simulink model "fbl_4wd_withCtrller"  (R2020b)
settings: Solver=VariableStepAuto  StartTime=0.0  StopTime=50  RelTol=1e-3
values from neighbouring files (symbols this model uses):
  a = 0.37    [main.m]
  b = 0.55    [main.m]
  d0 = 0.18    [main.m]
  fr_act = 0.12    [main.m]
  g = 9.81    [main.m]
  I = 20    [main.m]
  Ka1 = 0    [main.m]
  Ka2 = 0    [main.m]
  Kp1 = 60    [main.m]
  Kp2 = 60    [main.m]
  Kv1 = 40    [main.m]
  Kv2 = 40    [main.m]
  M = [m 0 0; 0 m 0; 0 0 I]    [main.m]
  m = 116    [main.m]
  mu_act = 0.88    [main.m]
  q0 = [0;0;deg2rad(10)]    [main.m]
  q0_dot = [[cos(q0(3)) -sin(q0(3));sin(q0(3)) cos(q0(3))]*[0.5;0.5];-2.2]    [main.m]
  r = 0.2    [main.m]
settings Model: Creator=sumit  LastModifiedBy=sumit
settings SolverCC: AlgebraicLoopSolver=LineSearch

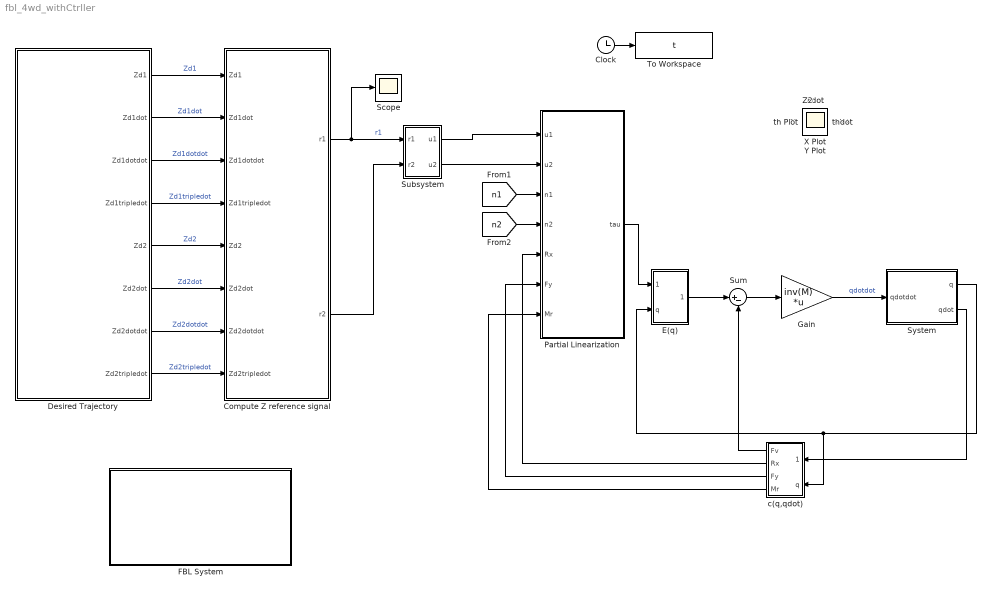
== system fbl_4wd_withCtrller ==
  Clock : Clock
  Compute Z reference signal : Subsystem
  Desired Trajectory : Subsystem
  E(q) : Subsystem
  FBL System : Subsystem
  Gain : Gain  Gain=inv(M)  Multiplication=Matrix(K*u)
  Partial Linearization : MATLAB Function  TreatAsAtomicUnit=on
      settings: MinAlgLoopOccurrences=on
  Scope : Scope
  Subsystem : Subsystem
  Sum : Sum  Inputs=|+-
  System : Subsystem
  To Workspace : ToWorkspace  VariableName=t  SampleTime=-1
  c(q,qdot) : Subsystem
  X Plot : Scope
  Xdot : Scope
  Y Plot : Scope
  Ydot : Scope
  Z1 : Scope
  Z2 : Scope
  th Plot : Scope
  thdot : Scope
  wires:
  Clock/1 -> To Workspace/1
  Sum/1 -> Gain/1
  c(q,qdot)/1(Fv) -> Sum/2
  E(q)/1(Ftau) -> Sum/1
  Partial Linearization/1(tau) -> E(q)/1(tau)
  c(q,qdot)/4(Mr) -> Partial Linearization/7(Mr)
  c(q,qdot)/3(Fy) -> Partial Linearization/6(Fy)
  c(q,qdot)/2(Rx) -> Partial Linearization/5(Rx)
  [n1] -> Partial Linearization/3(n1)
  [n2] -> Partial Linearization/4(n2)
  Desired Trajectory/1(Zd1) -> Compute Z reference signal/1(Zd1)  "Zd1"
  Desired Trajectory/2(Zd1dot) -> Compute Z reference signal/2(Zd1dot)  "Zd1dot"
  Desired Trajectory/3(Zd1dotdot) -> Compute Z reference signal/3(Zd1dotdot)  "Zd1dotdot"
  Desired Trajectory/4(Zd1tripledot) -> Compute Z reference signal/4(Zd1tripledot)  "Zd1tripledot"
  Desired Trajectory/5(Zd2) -> Compute Z reference signal/5(Zd2)  "Zd2"
  Desired Trajectory/6(Zd2dot) -> Compute Z reference signal/6(Zd2dot)  "Zd2dot"
  Desired Trajectory/7(Zd2dotdot) -> Compute Z reference signal/7(Zd2dotdot)  "Zd2dotdot"
  Desired Trajectory/8(Zd2tripledot) -> Compute Z reference signal/8(Zd2tripledot)  "Zd2tripledot"
  Compute Z reference signal/1(r1) -> Scope/1, Subsystem/1(r1)  "r1"
  Compute Z reference signal/2(r2) -> Subsystem/2(r2)
  Subsystem/1(u1) -> Partial Linearization/1(u1)
  Subsystem/2(u2) -> Partial Linearization/2(u2)
  System/1(q) -> c(q,qdot)/2(q), E(q)/2(q)
  Gain/1 -> System/1(qdotdot)  "qdotdot"
  System/2(qdot) -> c(q,qdot)/1(qdot)

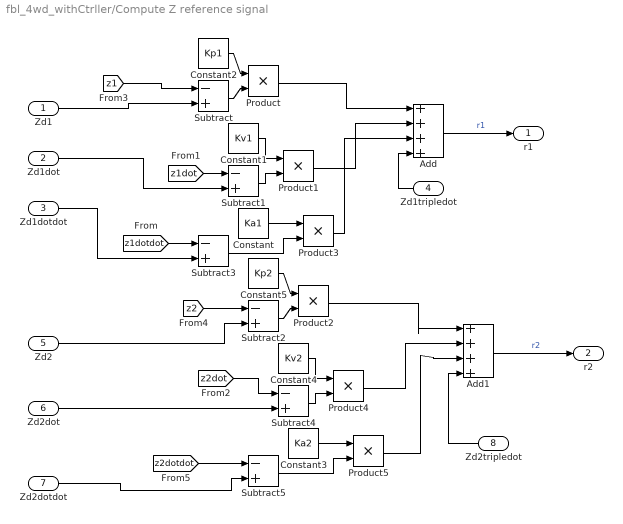
== system fbl_4wd_withCtrller/Compute Z reference signal ==
  Zd1 : Inport
  Zd1dot : Inport  Port=2
  Zd1dotdot : Inport  Port=3
  Zd1tripledot : Inport  Port=4
  Zd2 : Inport  Port=5
  Zd2dot : Inport  Port=6
  Zd2dotdot : Inport  Port=7
  Zd2tripledot : Inport  Port=8
  Add : Sum  Inputs=++++
  Add1 : Sum  Inputs=++++
  Constant : Constant  Value=Ka1
  Constant1 : Constant  Value=Kv1
  Constant2 : Constant  Value=Kp1
  Constant3 : Constant  Value=Ka2
  Constant4 : Constant  Value=Kv2
  Constant5 : Constant  Value=Kp2
  Product{,1..5} (6 alike) : Product
  Subtract{,1..5} (6 alike) : Sum  Inputs=-+
  r1 : Outport
  r2 : Outport  Port=2
  wires:
  Zd2dot/1 -> Subtract4/2
  Constant5/1 -> Product2/1
  [z2] -> Subtract2/1
  Product/1 -> Add/1
  Product3/1 -> Add/3
  Subtract1/1 -> Product1/2
  [z2dot] -> Subtract4/1
  Subtract4/1 -> Product4/2
  Subtract5/1 -> Product5/2
  Product5/1 -> Add1/3
  Constant2/1 -> Product/1
  Zd1/1 -> Subtract/2
  Product2/1 -> Add1/1
  Add1/1 -> r2/1  "r2"
  Product4/1 -> Add1/2
  Subtract3/1 -> Product3/2
  Constant4/1 -> Product4/1
  Constant3/1 -> Product5/1
  Add/1 -> r1/1  "r1"
  Subtract2/1 -> Product2/2
  [z1dot] -> Subtract1/1
  Constant1/1 -> Product1/1
  Zd1dot/1 -> Subtract1/2
  Constant/1 -> Product3/1
  Subtract/1 -> Product/2
  Product1/1 -> Add/2
  [z2dotdot] -> Subtract5/1
  Zd1tripledot/1 -> Add/4
  Zd1dotdot/1 -> Subtract3/2
  [z1] -> Subtract/1
  Zd2tripledot/1 -> Add1/4
  [z1dotdot] -> Subtract3/1
  Zd2dotdot/1 -> Subtract5/2
  Zd2/1 -> Subtract2/2

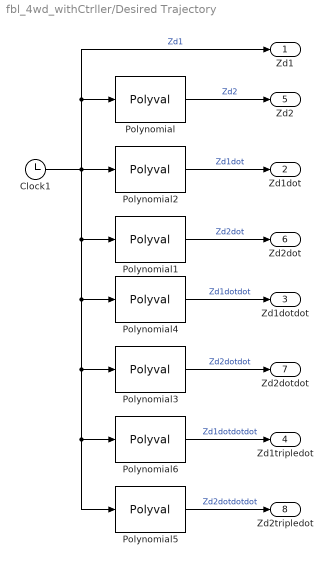
== system fbl_4wd_withCtrller/Desired Trajectory ==
  Clock1 : Clock
  Polynomial : Polyval  Coefs=[-0.002 0.1 0.1 0]
  Polynomial1 : Polyval  Coefs=[-0.006 0.2 0.1]
  Polynomial2 : Polyval  Coefs=[1]
  Polynomial3 : Polyval  Coefs=[-0.012 0.2]
  Polynomial4 : Polyval  Coefs=[0]
  Polynomial5 : Polyval  Coefs=[-0.012 0.2]
  Polynomial6 : Polyval  Coefs=[0]
  Zd1 : Outport
  Zd1dot : Outport  Port=2
  Zd1dotdot : Outport  Port=3
  Zd1tripledot : Outport  Port=4
  Zd2 : Outport  Port=5
  Zd2dot : Outport  Port=6
  Zd2dotdot : Outport  Port=7
  Zd2tripledot : Outport  Port=8
  wires:
  Polynomial/1 -> Zd2/1  "Zd2"
  Polynomial1/1 -> Zd2dot/1  "Zd2dot"
  Polynomial2/1 -> Zd1dot/1  "Zd1dot"
  Polynomial4/1 -> Zd1dotdot/1  "Zd1dotdot"
  Polynomial3/1 -> Zd2dotdot/1  "Zd2dotdot"
  Polynomial6/1 -> Zd1tripledot/1  "Zd1dotdotdot"
  Polynomial5/1 -> Zd2tripledot/1  "Zd2dotdotdot"
  Clock1/1 -> Polynomial6/1, Polynomial5/1, Polynomial3/1, Polynomial4/1, Polynomial1/1, Polynomial2/1, Zd1/1, Polynomial/1  "Zd1"

== system fbl_4wd_withCtrller/E(q) ==
  tau : Inport
  q : Inport  Port=2
  Demux : Demux  Outputs=3
  Eq : MATLAB Function  TreatAsAtomicUnit=on
      settings: MinAlgLoopOccurrences=on
  Terminator : Terminator
  Terminator1 : Terminator
  Ftau : Outport
  wires:
  Demux/1 -> Terminator/1
  Eq/1(Ftau) -> Ftau/1
  q/1 -> Demux/1
  Demux/2 -> Terminator1/1
  tau/1 -> Eq/1(tau)
  Demux/3 -> Eq/2(theta)

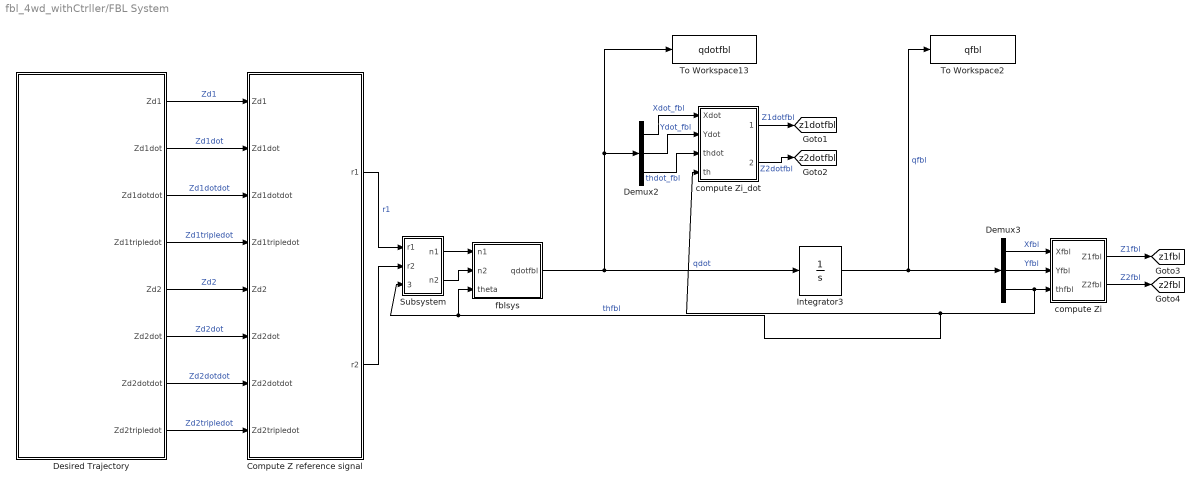
== system fbl_4wd_withCtrller/FBL System ==
  Compute Z reference signal : Subsystem
  Demux2 : Demux  Outputs=3
  Demux3 : Demux  Outputs=3
  Desired Trajectory : Subsystem
  Integrator3 : Integrator  InitialCondition=q0
  Subsystem : Subsystem
  To Workspace13 : ToWorkspace  VariableName=qdotfbl  SampleTime=-1
  To Workspace2 : ToWorkspace  VariableName=qfbl  SampleTime=-1
  compute Zi : Subsystem
  compute Zi_dot : Subsystem
  fblsys : MATLAB Function  TreatAsAtomicUnit=on
  tag scope: z1dotfbl=global, z1fbl=global, z2dotfbl=global, z2fbl=global
  wires:
  Integrator3/1 -> Demux3/1, To Workspace2/1  "qfbl"
  fblsys/1(qdotfbl) -> Integrator3/1, To Workspace13/1, Demux2/1  "qdot"
  Demux3/3 -> fblsys/3(theta), Subsystem/3(theta), compute Zi_dot/4(th), compute Zi/3(thfbl)  "thfbl"
  Demux2/1 -> compute Zi_dot/1(Xdot)  "Xdot_fbl"
  Demux2/3 -> compute Zi_dot/3(thdot)  "thdot_fbl"
  Demux2/2 -> compute Zi_dot/2(Ydot)  "Ydot_fbl"
  Demux3/1 -> compute Zi/1(Xfbl)  "Xfbl"
  Demux3/2 -> compute Zi/2(Yfbl)  "Yfbl"
  compute Zi/1(Z1fbl) -> [z1fbl]  "Z1fbl"
  compute Zi/2(Z2fbl) -> [z2fbl]  "Z2fbl"
  Desired Trajectory/2(Zd1dot) -> Compute Z reference signal/2(Zd1dot)  "Zd1dot"
  Desired Trajectory/7(Zd2dotdot) -> Compute Z reference signal/7(Zd2dotdot)  "Zd2dotdot"
  Desired Trajectory/6(Zd2dot) -> Compute Z reference signal/6(Zd2dot)  "Zd2dot"
  Desired Trajectory/3(Zd1dotdot) -> Compute Z reference signal/3(Zd1dotdot)  "Zd1dotdot"
  Desired Trajectory/5(Zd2) -> Compute Z reference signal/5(Zd2)  "Zd2"
  Desired Trajectory/8(Zd2tripledot) -> Compute Z reference signal/8(Zd2tripledot)  "Zd2tripledot"
  Desired Trajectory/4(Zd1tripledot) -> Compute Z reference signal/4(Zd1tripledot)  "Zd1tripledot"
  Desired Trajectory/1(Zd1) -> Compute Z reference signal/1(Zd1)  "Zd1"
  Compute Z reference signal/1(r1) -> Subsystem/1(r1)  "r1"
  Compute Z reference signal/2(r2) -> Subsystem/2(r2)
  Subsystem/2(n2) -> fblsys/2(n2)
  Subsystem/1(n1) -> fblsys/1(n1)
  compute Zi_dot/1(Z1dot) -> [z1dotfbl]  "Z1dotfbl"
  compute Zi_dot/2(Z2dot) -> [z2dotfbl]  "Z2dotfbl"

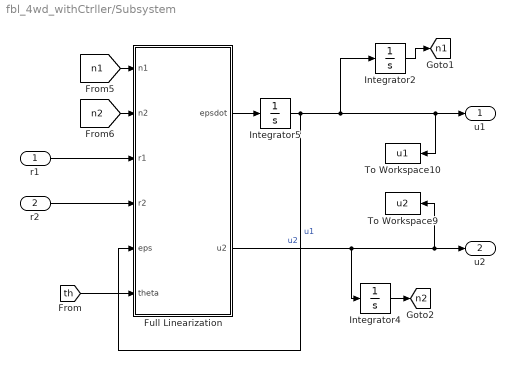
== system fbl_4wd_withCtrller/Subsystem ==
  r1 : Inport
  r2 : Inport  Port=2
  Full Linearization : MATLAB Function  TreatAsAtomicUnit=on
      settings: MinAlgLoopOccurrences=on
  Integrator2 : Integrator
  Integrator4 : Integrator
  Integrator5 : Integrator
  To Workspace10 : ToWorkspace  VariableName=u1  SampleTime=-1
  To Workspace9 : ToWorkspace  VariableName=u2  SampleTime=-1
  u1 : Outport
  u2 : Outport  Port=2
  tag scope: n1=global, n2=global
  wires:
  [n1] -> Full Linearization/1(n1)
  Full Linearization/1(epsdot) -> Integrator5/1
  Full Linearization/2(u2) -> Integrator4/1, To Workspace9/1, u2/1  "u2"
  Integrator5/1 -> Integrator2/1, u1/1, To Workspace10/1, Full Linearization/5(eps)  "u1"
  [n2] -> Full Linearization/2(n2)
  r1/1 -> Full Linearization/3(r1)
  Integrator2/1 -> [n1]
  Integrator4/1 -> [n2]
  [th] -> Full Linearization/6(theta)
  r2/1 -> Full Linearization/4(r2)

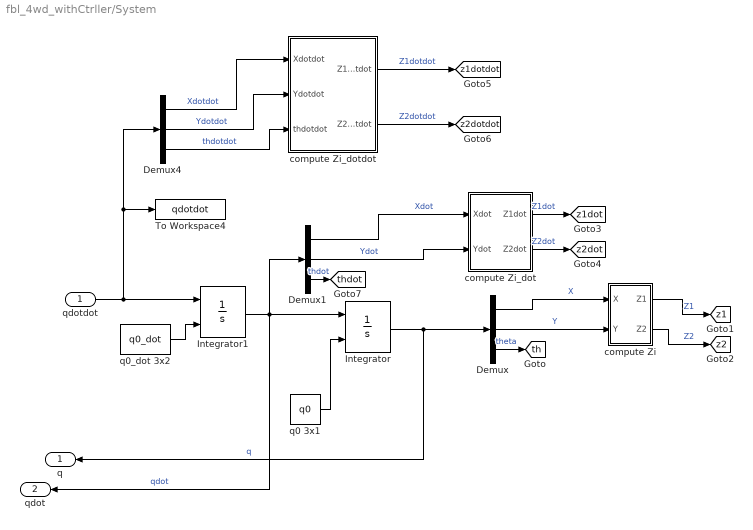
== system fbl_4wd_withCtrller/System ==
  qdotdot : Inport
  Demux : Demux  Outputs=3
  Demux1 : Demux  Outputs=3
  Demux4 : Demux  Outputs=3
  Integrator : Integrator  InitialConditionSource=external
  Integrator1 : Integrator  InitialConditionSource=external
  To Workspace4 : ToWorkspace  VariableName=qdotdot  SampleTime=-1
  compute Zi : Subsystem
  compute Zi_dot : Subsystem
  compute Zi_dotdot : Subsystem
  q0 3x1 : Constant  Value=q0
  q0_dot 3x2 : Constant  Value=q0_dot
  q : Outport
  qdot : Outport  Port=2
  tag scope: th=global, thdot=global, z1=global, z1dot=global, z1dotdot=global, z2=global, z2dot=global, z2dotdot=global
  wires:
  compute Zi_dot/2(Z2dot) -> [z2dot]  "Z2dot"
  Demux1/3 -> [thdot]  "thdot"
  Demux/3 -> [th]  "theta"
  Demux4/2 -> compute Zi_dotdot/2(Ydotdot)  "Ydotdot"
  qdotdot/1 -> Integrator1/1, Demux4/1, To Workspace4/1
  q0_dot 3x2/1 -> Integrator1/2
  Demux4/3 -> compute Zi_dotdot/3(thdotdot)  "thdotdot"
  compute Zi/2(Z2) -> [z2]  "Z2"
  q0 3x1/1 -> Integrator/2
  compute Zi_dotdot/1(Z1dotdot) -> [z1dotdot]  "Z1dotdot"
  Integrator/1 -> q/1, Demux/1  "q"
  Demux1/2 -> compute Zi_dot/2(Ydot)  "Ydot"
  Integrator1/1 -> qdot/1, Demux1/1, Integrator/1  "qdot"
  compute Zi_dotdot/2(Z2dotdot) -> [z2dotdot]  "Z2dotdot"
  compute Zi/1(Z1) -> [z1]  "Z1"
  Demux/1 -> compute Zi/1(X)  "X"
  Demux1/1 -> compute Zi_dot/1(Xdot)  "Xdot"
  Demux/2 -> compute Zi/2(Y)  "Y"
  compute Zi_dot/1(Z1dot) -> [z1dot]  "Z1dot"
  Demux4/1 -> compute Zi_dotdot/1(Xdotdot)  "Xdotdot"

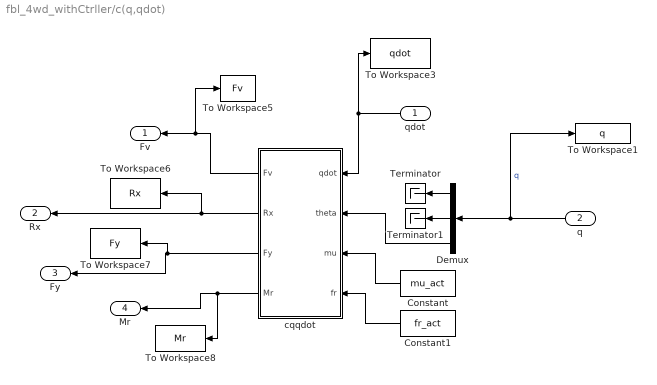
== system fbl_4wd_withCtrller/c(q,qdot) ==
  qdot : Inport
  q : Inport  Port=2
  Constant : Constant  Value=mu_act
  Constant1 : Constant  Value=fr_act
  Demux : Demux  Outputs=3
  Terminator : Terminator
  Terminator1 : Terminator
  To Workspace1 : ToWorkspace  VariableName=q  SampleTime=-1
  To Workspace3 : ToWorkspace  VariableName=qdot  SampleTime=-1
  To Workspace5 : ToWorkspace  VariableName=Fv  SampleTime=-1
  To Workspace6 : ToWorkspace  VariableName=Rx  SampleTime=-1
  To Workspace7 : ToWorkspace  VariableName=Fy  SampleTime=-1
  To Workspace8 : ToWorkspace  VariableName=Mr  SampleTime=-1
  cqqdot : MATLAB Function  TreatAsAtomicUnit=on
  Fv : Outport
  Rx : Outport  Port=2
  Fy : Outport  Port=3
  Mr : Outport  Port=4
  wires:
  Demux/2 -> Terminator1/1
  qdot/1 -> To Workspace3/1, cqqdot/1(qdot)
  Constant1/1 -> cqqdot/4(fr)
  Demux/1 -> Terminator/1
  Constant/1 -> cqqdot/3(mu)
  Demux/3 -> cqqdot/2(theta)
  cqqdot/3(Fy) -> To Workspace7/1, Fy/1
  cqqdot/2(Rx) -> To Workspace6/1, Rx/1
  cqqdot/4(Mr) -> To Workspace8/1, Mr/1
  cqqdot/1(Fv) -> To Workspace5/1, Fv/1
  q/1 -> To Workspace1/1, Demux/1  "q"

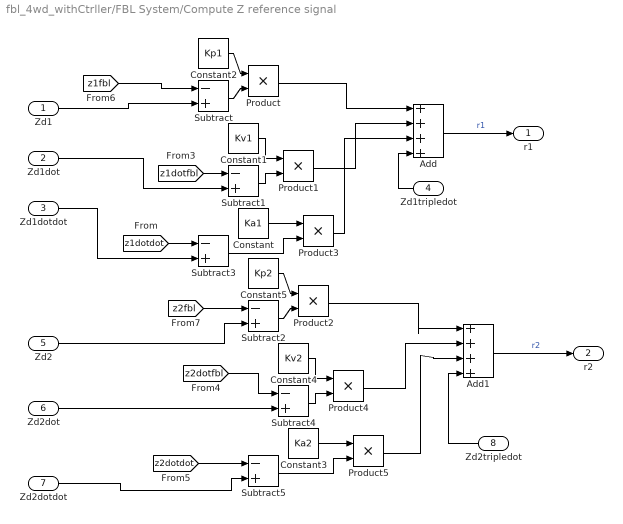
== system fbl_4wd_withCtrller/FBL System/Compute Z reference signal ==
  Zd1 : Inport
  Zd1dot : Inport  Port=2
  Zd1dotdot : Inport  Port=3
  Zd1tripledot : Inport  Port=4
  Zd2 : Inport  Port=5
  Zd2dot : Inport  Port=6
  Zd2dotdot : Inport  Port=7
  Zd2tripledot : Inport  Port=8
  Add : Sum  Inputs=++++
  Add1 : Sum  Inputs=++++
  Constant : Constant  Value=Ka1
  Constant1 : Constant  Value=Kv1
  Constant2 : Constant  Value=Kp1
  Constant3 : Constant  Value=Ka2
  Constant4 : Constant  Value=Kv2
  Constant5 : Constant  Value=Kp2
  Product{,1..5} (6 alike) : Product
  Subtract{,1..5} (6 alike) : Sum  Inputs=-+
  r1 : Outport
  r2 : Outport  Port=2
  wires:
  Zd2dot/1 -> Subtract4/2
  Constant5/1 -> Product2/1
  [z2fbl] -> Subtract2/1
  Product/1 -> Add/1
  Product3/1 -> Add/3
  Subtract1/1 -> Product1/2
  [z2dotfbl] -> Subtract4/1
  Subtract4/1 -> Product4/2
  Subtract5/1 -> Product5/2
  Product5/1 -> Add1/3
  Constant2/1 -> Product/1
  Zd1/1 -> Subtract/2
  Product2/1 -> Add1/1
  Add1/1 -> r2/1  "r2"
  Product4/1 -> Add1/2
  Subtract3/1 -> Product3/2
  Constant4/1 -> Product4/1
  Constant3/1 -> Product5/1
  Add/1 -> r1/1  "r1"
  Subtract2/1 -> Product2/2
  [z1dotfbl] -> Subtract1/1
  Constant1/1 -> Product1/1
  Zd1dot/1 -> Subtract1/2
  Constant/1 -> Product3/1
  Subtract/1 -> Product/2
  Product1/1 -> Add/2
  [z2dotdot] -> Subtract5/1
  Zd1tripledot/1 -> Add/4
  Zd1dotdot/1 -> Subtract3/2
  [z1fbl] -> Subtract/1
  Zd2tripledot/1 -> Add1/4
  [z1dotdot] -> Subtract3/1
  Zd2dotdot/1 -> Subtract5/2
  Zd2/1 -> Subtract2/2

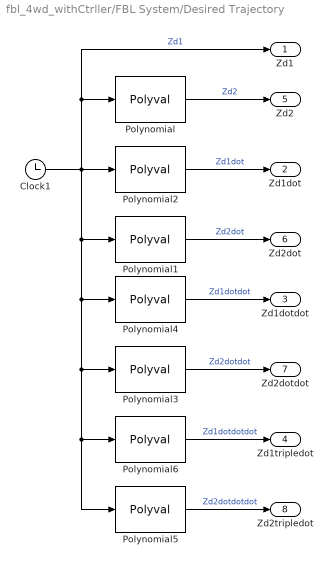
== system fbl_4wd_withCtrller/FBL System/Desired Trajectory ==
  Clock1 : Clock
  Polynomial : Polyval  Coefs=[-0.002 0.1 0.1 0]
  Polynomial1 : Polyval  Coefs=[-0.006 0.2 0.1]
  Polynomial2 : Polyval  Coefs=[1]
  Polynomial3 : Polyval  Coefs=[-0.012 0.2]
  Polynomial4 : Polyval  Coefs=[0]
  Polynomial5 : Polyval  Coefs=[-0.012 0.2]
  Polynomial6 : Polyval  Coefs=[0]
  Zd1 : Outport
  Zd1dot : Outport  Port=2
  Zd1dotdot : Outport  Port=3
  Zd1tripledot : Outport  Port=4
  Zd2 : Outport  Port=5
  Zd2dot : Outport  Port=6
  Zd2dotdot : Outport  Port=7
  Zd2tripledot : Outport  Port=8
  wires:
  Polynomial/1 -> Zd2/1  "Zd2"
  Polynomial1/1 -> Zd2dot/1  "Zd2dot"
  Polynomial2/1 -> Zd1dot/1  "Zd1dot"
  Polynomial4/1 -> Zd1dotdot/1  "Zd1dotdot"
  Polynomial3/1 -> Zd2dotdot/1  "Zd2dotdot"
  Polynomial6/1 -> Zd1tripledot/1  "Zd1dotdotdot"
  Polynomial5/1 -> Zd2tripledot/1  "Zd2dotdotdot"
  Clock1/1 -> Polynomial6/1, Polynomial5/1, Polynomial3/1, Polynomial4/1, Polynomial1/1, Polynomial2/1, Zd1/1, Polynomial/1  "Zd1"

== system fbl_4wd_withCtrller/FBL System/Subsystem ==
  r1 : Inport
  r2 : Inport  Port=2
  theta : Inport  Port=3
  Full Linearization : MATLAB Function  TreatAsAtomicUnit=on
      settings: MinAlgLoopOccurrences=on
  Integrator2 : Integrator
  Integrator4 : Integrator
  Integrator5 : Integrator
  To Workspace1 : ToWorkspace  VariableName=n1fbl  SampleTime=-1
  To Workspace10 : ToWorkspace  VariableName=u1fbl  SampleTime=-1
  To Workspace2 : ToWorkspace  VariableName=n2fbl  SampleTime=-1
  To Workspace9 : ToWorkspace  VariableName=u2fbl  SampleTime=-1
  n1 : Outport
  n2 : Outport  Port=2
  wires:
  Integrator2/1 -> To Workspace1/1, Full Linearization/1(n1), n1/1
  Full Linearization/1(epsdot) -> Integrator5/1
  Full Linearization/2(u2) -> Integrator4/1, To Workspace9/1  "u2"
  Integrator5/1 -> Integrator2/1, To Workspace10/1, Full Linearization/5(eps)  "u1"
  Integrator4/1 -> To Workspace2/1, Full Linearization/2(n2), n2/1
  r1/1 -> Full Linearization/3(r1)
  theta/1 -> Full Linearization/6(theta)
  r2/1 -> Full Linearization/4(r2)

== system fbl_4wd_withCtrller/FBL System/compute Zi ==
  Xfbl : Inport
  Yfbl : Inport  Port=2
  thfbl : Inport  Port=3
  Constant : Constant  Value=d0
  Constant1 : Constant  Value=d0
  Cos : Trigonometry  Operator=cos
  Cos1 : Trigonometry
  Product : Product
  Product1 : Product
  Sum1 : Sum
  Sum2 : Sum
  Z1fbl : Outport
  Z2fbl : Outport  Port=2
  wires:
  Product1/1 -> Sum2/2
  Cos1/1 -> Product1/1
  Cos/1 -> Product/1
  Xfbl/1 -> Sum1/1
  Constant1/1 -> Product1/2
  thfbl/1 -> Cos1/1, Cos/1
  Product/1 -> Sum1/2
  Constant/1 -> Product/2
  Yfbl/1 -> Sum2/1
  Sum1/1 -> Z1fbl/1  "Z1fbl"
  Sum2/1 -> Z2fbl/1  "Z2fbl"

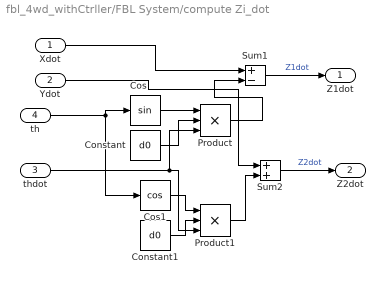
== system fbl_4wd_withCtrller/FBL System/compute Zi_dot ==
  Xdot : Inport
  Ydot : Inport  Port=2
  thdot : Inport  Port=3
  th : Inport  Port=4
  Constant : Constant  Value=d0
  Constant1 : Constant  Value=d0
  Cos : Trigonometry
  Cos1 : Trigonometry  Operator=cos
  Product : Product  Inputs=3
  Product1 : Product  Inputs=3
  Sum1 : Sum  Inputs=+-
  Sum2 : Sum
  Z1dot : Outport
  Z2dot : Outport  Port=2
  wires:
  Product1/1 -> Sum2/2
  Cos1/1 -> Product1/1
  Cos/1 -> Product/1
  Xdot/1 -> Sum1/1
  Constant1/1 -> Product1/2
  th/1 -> Cos1/1, Cos/1
  Product/1 -> Sum1/2
  Constant/1 -> Product/2
  Ydot/1 -> Sum2/1
  Sum1/1 -> Z1dot/1  "Z1dot"
  Sum2/1 -> Z2dot/1  "Z2dot"
  thdot/1 -> Product/3, Product1/3

== system fbl_4wd_withCtrller/System/compute Zi ==
  X : Inport
  Y : Inport  Port=2
  Constant : Constant  Value=d0
  Constant1 : Constant  Value=d0
  Cos : Trigonometry  Operator=cos
  Cos1 : Trigonometry
  Product : Product
  Product1 : Product
  Sum1 : Sum
  Sum2 : Sum
  Z1 : Outport
  Z2 : Outport  Port=2
  wires:
  Product1/1 -> Sum2/2
  Cos1/1 -> Product1/1
  Cos/1 -> Product/1
  X/1 -> Sum1/1
  Constant1/1 -> Product1/2
  [th] -> Cos/1, Cos1/1
  Product/1 -> Sum1/2
  Constant/1 -> Product/2
  Y/1 -> Sum2/1
  Sum1/1 -> Z1/1  "Z1"
  Sum2/1 -> Z2/1  "Z2"

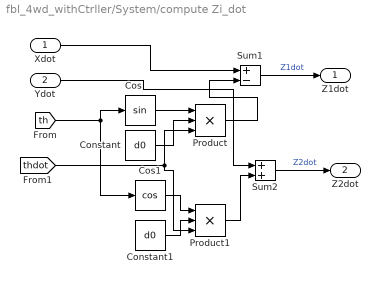
== system fbl_4wd_withCtrller/System/compute Zi_dot ==
  Xdot : Inport
  Ydot : Inport  Port=2
  Constant : Constant  Value=d0
  Constant1 : Constant  Value=d0
  Cos : Trigonometry
  Cos1 : Trigonometry  Operator=cos
  Product : Product  Inputs=3
  Product1 : Product  Inputs=3
  Sum1 : Sum  Inputs=+-
  Sum2 : Sum
  Z1dot : Outport
  Z2dot : Outport  Port=2
  wires:
  Product1/1 -> Sum2/2
  Cos1/1 -> Product1/1
  Cos/1 -> Product/1
  Xdot/1 -> Sum1/1
  Constant1/1 -> Product1/2
  [th] -> Cos/1, Cos1/1
  Product/1 -> Sum1/2
  Constant/1 -> Product/2
  Ydot/1 -> Sum2/1
  Sum1/1 -> Z1dot/1  "Z1dot"
  Sum2/1 -> Z2dot/1  "Z2dot"
  [thdot] -> Product1/3, Product/3

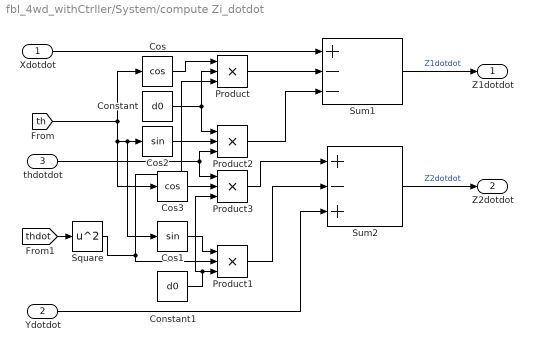
== system fbl_4wd_withCtrller/System/compute Zi_dotdot ==
  Xdotdot : Inport
  Ydotdot : Inport  Port=2
  thdotdot : Inport  Port=3
  Constant : Constant  Value=d0
  Constant1 : Constant  Value=d0
  Cos : Trigonometry  Operator=cos
  Cos1 : Trigonometry
  Cos2 : Trigonometry
  Cos3 : Trigonometry  Operator=cos
  Product{,1..3} (4 alike) : Product  Inputs=3
  Square : Math  Operator=square  SaturateOnIntegerOverflow=on
  Sum1 : Sum  Inputs=+--
  Sum2 : Sum  Inputs=+-+
  Z1dotdot : Outport
  Z2dotdot : Outport  Port=2
  wires:
  Product1/1 -> Sum2/2
  Cos1/1 -> Product1/1
  Cos/1 -> Product/1
  Xdotdot/1 -> Sum1/1
  [th] -> Cos3/1, Cos2/1, Cos1/1, Cos/1
  Product/1 -> Sum1/2
  Constant/1 -> Product2/1, Product/2
  Sum1/1 -> Z1dotdot/1  "Z1dotdot"
  Sum2/1 -> Z2dotdot/1  "Z2dotdot"
  [thdot] -> Square/1
  Square/1 -> Product/3, Product1/2
  Cos2/1 -> Product2/2
  thdotdot/1 -> Product3/1, Product2/3
  Ydotdot/1 -> Sum2/3
  Constant1/1 -> Product3/3, Product1/3
  Product2/1 -> Sum1/3
  Product3/1 -> Sum2/1
  Cos3/1 -> Product3/2

== matlab function fbl_4wd_withCtrller/E(q)/Eq ==
  data: tau input; theta input; Ftau output; t parameter; r parameter
function Ftau = Eq(tau,theta,t, r)
Ftau=[cos(theta)/r cos(theta)/r;...
   sin(theta)/r sin(theta)/r;...
   -t/r t/r]*tau;

== matlab function fbl_4wd_withCtrller/c(q,qdot)/cqqdot ==
  data: qdot input; theta input; Fv output; mu input; fr input; a parameter; b parameter; t parameter; g parameter; m parameter; Rx output; Fy output; Mr output
function [Fv,Rx,Fy,Mr] = cqqdot(qdot,theta,mu,fr,a, b, t, g, m)
Xdot=qdot(1);
Ydot=qdot(2);
thdot=qdot(3);

%Rth = [cos(theta) -sin(theta);sin(theta) cos(theta)];

xdot =  Xdot*cos(theta)+Ydot*sin(theta);
ydot = -Xdot*sin(theta)+Ydot*cos(theta);

x1dot = xdot-t*thdot;   
x2dot = xdot+t*thdot;
y1dot = ydot+a*thdot;
y3dot = ydot-b*thdot;

Rx = fr*m*g*0.5*(sign(x1dot)+sign(x2dot));
Fy = mu*m*g*(b*sign(y1dot)+a*sign(y3dot))/(a+b);
Mr = mu*a*b*m*g*(sign(y1dot)-sign(y3dot))/(a+b)...
     + fr*t*m*g*0.5*(sign(x2dot)-sign(x1dot));
 
Fv=[Rx*cos(theta)-Fy*sin(theta);...
   Rx*sin(theta)+Fy*cos(theta);...
   Mr];

== matlab function fbl_4wd_withCtrller/Partial Linearization ==
  data: u1 input; u2 input; n1 input; n2 input; Rx input; Fy input; Mr input; tau output; t parameter; r parameter; d0 parameter; m parameter; I parameter
function tau = FBL(u1,u2,n1,n2,Rx,Fy,Mr,t, r,d0, m, I)
tau=[r*0.5*(m*u1+m*n2*n2/d0+Rx)+(r*d0*0.5/t)*((m+I/(d0^2))*u2-m*n1*n2/d0...
    +Fy-Mr/d0);
     r*0.5*(m*u1+m*n2*n2/d0+Rx)-(r*d0*0.5/t)*((m+I/(d0^2))*u2-m*n1*n2/d0...
    +Fy-Mr/d0)];

== matlab function fbl_4wd_withCtrller/FBL System/fblsys ==
  data: n1 input; n2 input; theta input; qdotfbl output; d0 parameter
function qdotfbl = fblsys(n1, n2,theta,d0)
qdotfbl=[cos(theta)*n1-sin(theta)*n2;...
         sin(theta)*n1+cos(theta)*n2;...
         -n2/d0];

== matlab function fbl_4wd_withCtrller/Subsystem/Full Linearization ==
  data: n1 input; n2 input; d0 parameter; r1 input; r2 input; eps input; theta input; epsdot output; u2 output
function [epsdot,u2] = fulllin(n1,n2,d0,r1,r2, eps,theta)
epsdot = cos(theta)*r1+sin(theta)*r2+n1*n2*n2/(d0^2);
if round(n1)==0
    u2=0;
else
u2 = (sin(theta)*r1-cos(theta)*r2)*d0/n1-2*eps*n2/n1;
end

== matlab function fbl_4wd_withCtrller/FBL System/Subsystem/Full Linearization ==
  data: n1 input; n2 input; d0 parameter; r1 input; r2 input; eps input; theta input; epsdot output; u2 output
function [epsdot,u2] = fulllin(n1,n2,d0,r1,r2, eps,theta)
epsdot = cos(theta)*r1+sin(theta)*r2+n1*n2*n2/(d0^2);
if n1<1e-5
    u2=0;
else
u2 = (sin(theta)*r1-cos(theta)*r2)*d0/n1-2*eps*n2/n1;
end
